simulink model "final_lqr_integral_nonlinear_simulation"  (R2024a)
settings: Solver=VariableStepAuto  StartTime=0.0  StopTime=10.0  RelTol=1e-3
undefined symbols (not defined in the file): g_val, Ki, Kx, m_val, r_pos
libraries: slpidlib x1
settings Model: Creator=yufon  LastModifiedBy=yufon

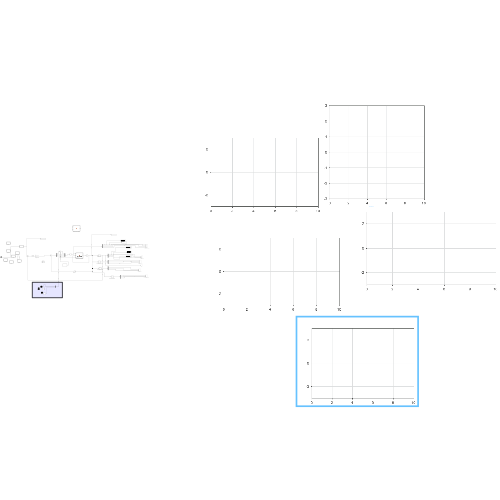
[thumbnail: Simulink's stored preview of the top-level diagram]
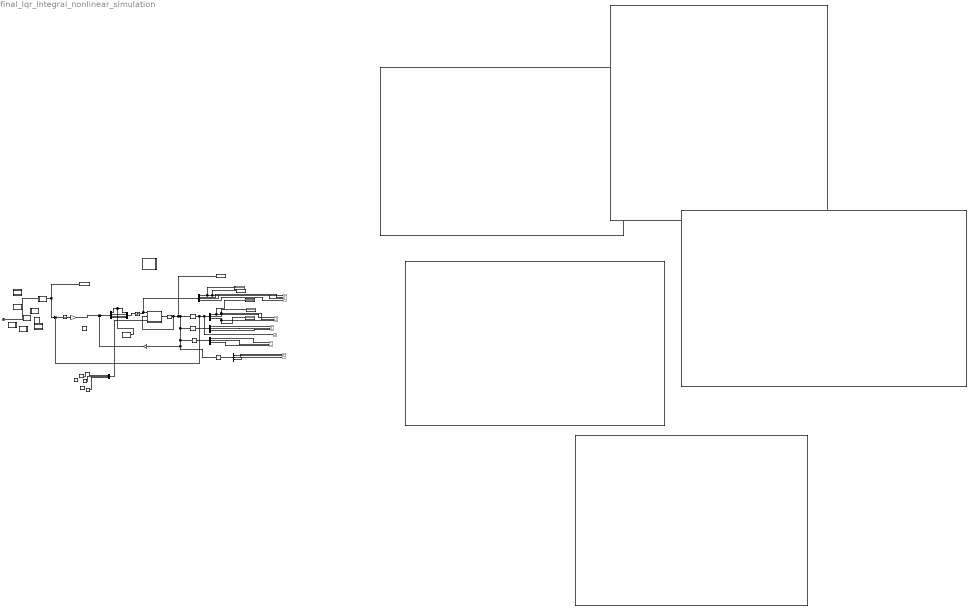
== system final_lqr_integral_nonlinear_simulation ==
  note: Wind Purtubabtions
  Arc : MATLAB Function  TreatAsAtomicUnit=on
  Body Abgular Selector : Selector  InputPortWidth=12  IndexOptions=Index vector (dialog)  Indices=[10 11 12]  OutputSizes=1
  Body Abgular Selector1 : Selector  InputPortWidth=12  IndexOptions=Index vector (dialog)  Indices=[7 8 9]  OutputSizes=1
  Body Linear Velocities : Scope  Commented=on  NumInputPorts=3
  Circular Trajectory : MATLAB Function  TreatAsAtomicUnit=on
  Clock : Clock
  Constant1 : Constant  Value=r_pos  VectorParams1D=off
  Constant2 : Constant  Value=m_val*g_val
  Constant4 : Constant  Value=0
  Constant5 : Constant  Value=0
  Control Input Scope : Scope  Commented=on  NumInputPorts=4
  Dashboard Scope{,1..4} (5 alike) : DashboardScope
  Demux{,1,3,5} (4 alike) : Demux  Outputs=3
  Demux2 : Demux
  Demux6 : Demux
  Display{,1..3} (4 alike) : Display
  Figure 8 : MATLAB Function  TreatAsAtomicUnit=on
  Helical : MATLAB Function  TreatAsAtomicUnit=on
  Integrator Gain : Gain  Gain=Ki  Multiplication=Matrix(K*u)
  Integrator4 : Integrator  InitialCondition=[0; 0; 0; zeros(9,1)]
  Integrator5 : Integrator
  LQR Gain : Gain  Gain=Kx  Multiplication=Matrix(K*u)
  Line : MATLAB Function  TreatAsAtomicUnit=on
  MATLAB Function1 : MATLAB Function  TreatAsAtomicUnit=on
  Mux2 : Mux
  Mux3 : Mux  Inputs=3
  Orientation Scope : Scope  Commented=on  NumInputPorts=3
  Orientation Selector1 : Selector  InputPortWidth=12  IndexOptions=Index vector (dialog)  Indices=[4 5 6]  OutputSizes=1
  PID Controller : slpidlib/PID Controller  Controller=PID  Form=Parallel  TimeDomain=Continuous-time  UseExternalTs=off  SampleTime=-1  IntegratorMethod=Forward Euler  FilterMethod=Forward Euler  ControllerParametersSource=internal  P=1  I=1  UseKiTs=off  D=0  UseExternalDerivativeSource=off  N=100  UseFilter=on  TunerSelectOption=Transfer Function Based (PID Tuner App)  InitialConditionSource=internal  InitialConditionForIntegrator=0  InitialConditionForFilter=0  DifferentiatorICPrevScaledInput=0  ExternalReset=none  TrackingMode=off  Kt=1  LimitOutput=off  SatLimitsSource=internal  UpperSaturationLimit=inf  LowerSaturationLimit=-inf  LinearizeAsGain=on  AntiWindupMode=none  Kb=1  LimitIntegrator=off  UpperIntegratorSaturationLimit=inf  LowerIntegratorSaturationLimit=-inf  POutMin=[]  POutMax=[]  IOutMin=[]  IOutMax=[]  DOutMin=[]  DOutMax=[]  NOutMin=[]  NOutMax=[]  SumOutMin=[]  SumOutMax=[]  SaturationOutMin=[]  SaturationOutMax=[]  PParamMin=[]  PParamMax=[]  IParamMin=[]  IParamMax=[]  DParamMin=[]  DParamMax=[]  NParamMin=[]  NParamMax=[]  KbParamMin=[]  KbParamMax=[]  KtParamMin=[]  KtParamMax=[]  KbOutMin=[]  KbOutMax=[]  KtOutMin=[]  KtOutMax=[]  IntegratorOutMin=[]  IntegratorOutMax=[]  FilterOutMin=[]  FilterOutMax=[]  SumI1OutMin=[]  SumI1OutMax=[]  SumI2OutMin=[]  SumI2OutMax=[]  SumI3OutMin=[]  SumI3OutMax=[]  SumI4OutMin=[]  SumI4OutMax=[]  SumDOutMin=[]  SumDOutMax=[]  DifferentiatorOutMin=[]  DifferentiatorOutMax=[]  FilterDiffOutCoefMin=[]  FilterDiffOutCoefMax=[]  ReciprocalOutMin=[]  ReciprocalOutMax=[]  SumDenOutMin=[]  SumDenOutMax=[]  SumNumOutMin=[]  SumNumOutMax=[]  DivideOutMin=[]  DivideOutMax=[]  UdiffTsProdOutMin=[]  UdiffTsProdOutMax=[]  NTsProdOutMin=[]  NTsProdOutMax=[]  UintegralTsProdOutMin=[]  UintegralTsProdOutMax=[]  UngainTsProdOutMin=[]  UngainTsProdOutMax=[]  ClampingZeroOutDataTypeStr=Inherit: Inherit via back propagation  ClampingZeroOutMin=[]  ClampingZeroOutMax=[]  FilterDenConstantOutDataTypeStr=Inherit: Inherit via back propagation  FilterDenConstantOutMin=[]  FilterDenConstantOutMax=[]  PCopyOutDataTypeStr=Inherit: Inherit via back propagation  PCopyOutMin=[]  PCopyOutMax=[]  NCopyOutDataTypeStr=Inherit: Inherit via back propagation  NCopyOutMin=[]  NCopyOutMax=[]  IntegratorContinuousStateAttributes=''  IntegratorStateMustResolveToSignalObject=off  IntegratorRTWStateStorageClass=Auto  FilterContinuousStateAttributes=''  FilterStateMustResolveToSignalObject=off  FilterRTWStateStorageClass=Auto  ParallelPVariant=InternalParameters  IdealPVariant=Disabled  IVariant=InternalParameters  DVariant=InternalParameters  IntegratorVariant=Continuous  SatVariant=Disabled  AWVariant=Passthrough  PCopyVariant=Disabled  TRVariant=Disabled  FdbkBlocksVariant=Forward  IdealPFdbkVariant=Disabled  SatFdbkVariant=Disabled  DerivativeFilterVariant=ContFilter  NVariant=InternalParameters  NCopyVariant=Disabled  FilterICVariant=InternalICsFilter  IntegratorICVariant=InternalICs  ExternalResetVariant=Disabled  TRSumVariant=Passthrough  SumFdbkVariant=Disabled  SumVariant=Sum_PID  TsampFilterVariant=InternalTs  TsampNgainVariant=Passthrough  TsampIntegralVariant=Disabled_SignalSpec  ExternalSaturationOutDataTypeStr=Inherit: Same as second input  DerivativeSourceVariant=ErrorSignal
  Position Scope : Scope  Commented=on  NumInputPorts=3
  Position Scope1 : Scope  Commented=on  NumInputPorts=3
  Position Selector : Selector  InputPortWidth=12  IndexOptions=Index vector (dialog)  Indices=[1 2 3]  OutputSizes=1
  Pulse Generator1 : DiscretePulseGenerator  Amplitude=10  Period=10  PulseWidth=5  PhaseDelay=20  SampleTime=10
  Pulse Generator3 : DiscretePulseGenerator  PulseType=Time based  Amplitude=3  Period=5  PhaseDelay=100
  Pulse Generator4 : DiscretePulseGenerator  PulseType=Time based  Amplitude=3  Period=10  PulseWidth=5  PhaseDelay=50
  Quadrotor Nonlinear Model1 : MATLAB Function  TreatAsAtomicUnit=on
  Quadrotor Nonlinear Model2 : MATLAB Function  TreatAsAtomicUnit=on
  Saturation1 : Saturate  UpperLimit=[40; 0.15; 0.1;0.1]  LowerLimit=[0; -0.15; -0.10; -0.10]
  Scope : Scope  Commented=on
  Simusoidal : MATLAB Function  TreatAsAtomicUnit=on
  Spiral : MATLAB Function  TreatAsAtomicUnit=on
  Sum : Sum  Inputs=|--
  Sum1 : Sum  Inputs=|+-
  Sum3 : Sum  Inputs=|++
  To Workspace : ToWorkspace  VariableName=X_states  SampleTime=-1
  To Workspace1 : ToWorkspace  VariableName=U1  SaveFormat=Timeseries  SampleTime=-1
  To Workspace2 : ToWorkspace  VariableName=r_traj  SaveFormat=Timeseries  SampleTime=-1
  wires:
  Constant4/1 -> Mux3/2
  Demux3/1 -> Position Scope1/1  "p"
  Saturation1/1 -> Demux2/1, Quadrotor Nonlinear Model1/1(u)
  Orientation Selector1/1 -> Demux1/1
  Pulse Generator4/1 -> Mux3/1
  Demux1/1 -> Orientation Scope/1  "Phi"
  Clock/1 -> MATLAB Function1/1(t)
  Constant5/1 -> Mux3/3
  Demux5/3 -> Body Linear Velocities/3  "w"
  Demux1/2 -> Orientation Scope/2  "Thata"
  Integrator Gain/1 -> Sum/1
  Sum1/1 -> Integrator5/1
  Demux6/1 -> Sum3/1  "U1"
  Sum3/1 -> Mux2/1
  Quadrotor Nonlinear Model1/1(dx) -> Integrator4/1  "X_states"
  Demux/3 -> Display1/1, Position Scope/3  "Z"
  Demux3/2 -> Position Scope1/2  "q"
  Demux2/1 -> Display3/1, To Workspace1/1, Control Input Scope/1  "U1"
  Demux1/3 -> Orientation Scope/3  "Psi"
  Demux3/3 -> Position Scope1/3  "r"
  MATLAB Function1/1(r) -> To Workspace2/1, Sum1/1
  Demux/1 -> Display2/1, Position Scope/1  "X"
  Demux6/3 -> Mux2/3  "U3"
  Integrator4/1 -> To Workspace/1, Body Abgular Selector1/1, LQR Gain/1, Body Abgular Selector/1, Orientation Selector1/1, Position Selector/1, Quadrotor Nonlinear Model1/2(x)
  Mux3/1 -> Quadrotor Nonlinear Model1/3(F_wind_body)
  Demux2/2 -> Control Input Scope/2  "U2"
  Body Abgular Selector/1 -> Demux3/1
  Demux2/3 -> Control Input Scope/3  "U3"
  Position Selector/1 -> Scope/1, Demux/1, Sum1/2
  Demux6/4 -> Mux2/4  "U4"
  Mux2/1 -> Saturation1/1
  Constant2/1 -> Sum3/2
  Demux/2 -> Display/1, Position Scope/2  "Y"
  LQR Gain/1 -> Sum/2
  Demux2/4 -> Control Input Scope/4  "U4"
  Demux5/2 -> Body Linear Velocities/2  "u"
  Demux6/2 -> Mux2/2  "U2"
  Body Abgular Selector1/1 -> Demux5/1
  Integrator5/1 -> Integrator Gain/1
  Sum/1 -> Demux6/1
  Demux5/1 -> Body Linear Velocities/1  "u"

== matlab function final_lqr_integral_nonlinear_simulation/Line ==
  data: t input; r output
function r = linear_ref(t)
    % Define total time and start/end positions
    T_total = 50;  % duration of trajectory
    r_start = [0; 0; 0];
    r_end   = [5; 5; 5];

    % Clamp progress between 0 and 1
    progress = min(max(t / T_total, 0), 1);

    % Linear interpolation
    r = r_start + (r_end - r_start) * progress;
end

== matlab function final_lqr_integral_nonlinear_simulation/MATLAB Function1 ==
  data: t input; r output
function r = rectangular_trajectory(t)
    % Rectangular trajectory parameters
    x_length = 10;       % Rectangle length (x-direction) in meters
    y_width = 8;         % Rectangle width (y-direction) in meters
    z_height = 5;        % Z height in meters
    duration = 500;       % Total duration in seconds
    
    % Add initial offset to match quadcopter starting position
    x_offset = 0;        % Starting at x=0
    y_offset = 0;        % Starting at y=0
    z_offset = 0;        % Starting at z=0
    
    % Time progression (clamped between 0 and 1)
    progress = min(max(t / duration, 0), 1);
    
    % Define the four segments of the rectangle
    % Each segment takes 25% of the total time
    if progress < 0.25 
        % First segment: Moving along x-axis (0 to x_length)
        segment_progress = progress / 0.25;
        x_ref = x_offset + x_length * segment_progress;
        y_ref = y_offset;
        z_ref = z_offset + z_height * segment_progress;
    elseif progress < 0.5
        % Second segment: Moving along y-axis (0 to y_width)
        segment_progress = (progress - 0.25) / 0.25;
        x_ref = x_offset + x_length;
        y_ref = y_offset + y_width * segment_progress;
        z_ref = z_offset + z_height;
    elseif progress < 0.75
        % Third segment: Moving along x-axis (x_length to 0)
        segment_progress = (progress - 0.5) / 0.25;
        x_ref = x_offset + x_length * (1 - segment_progress);
        y_ref = y_offset + y_width;
        z_ref = z_offset + z_height;
    else
        % Fourth segment: Moving along y-axis (y_width to 0)
        segment_progress = (progress - 0.75) / 0.25;
        x_ref = x_offset;
        y_ref = y_offset + y_width * (1 - segment_progress);
        z_ref = z_offset + z_height;
    end
    
    r = [x_ref; y_ref; z_ref];
end

== matlab function final_lqr_integral_nonlinear_simulation/Quadrotor Nonlinear Model1 ==
  data: u input size=[4 1]; x input size=[12 1]; dx output size=[12 1]; F_wind_body input
function dx = quadrotor_dynamics(u, x, F_wind_body)
    % Physical parameters
    m = 0.547; % Mass [kg]
    g = 9.81; % Gravity [m/s^2]
    Cd = 1.0; % Drag coefficient [-]
    Ix = 3.3e-3;
    Iy = 3.3e-3;
    Iz = 5.8e-3;
    Ax = 0.011;
    Ay = 0.011;
    Az = 0.022;
    rho = 1.225; % Air density [kg/m^3]
    
    % REMOVE THIS LINE - it overwrites the input state!
    % x = zeros(12,1);
    
    % State unpacking
    phi = x(4); theta = x(5); psi = x(6);
    u_b = x(7); v_b = x(8); w_b = x(9);
    p = x(10); q = x(11); r = x(12);


    % Compute wind acceleration
    a_wind_body = F_wind_body / m;
    
    % Input unpacking with saturation
    U1 = max(0, min(30*m*g, u(1))); % Limit thrust to reasonable bounds
    U2 = max(-10, min(10, u(2)));   % Limit torques
    U3 = max(-10, min(10, u(3)));
    U4 = max(-10, min(10, u(4)));
    
    % Trig functions
    s = @sin; c = @cos; t = @tan;
    
    % Safety factor to prevent division by zero or extreme values
    eps = 1e-4;
    safe_cos_theta = max(eps, abs(cos(theta)));
    
    dx = zeros(12,1);
    
    % Translational Kinematics (Inertial frame)
    dx(1) = u_b*(c(theta)*c(psi)) + v_b*(s(phi)*s(theta)*c(psi) - c(phi)*s(psi)) + w_b*(c(phi)*s(theta)*c(psi) + s(phi)*s(psi));
    dx(2) = u_b*(c(theta)*s(psi)) + v_b*(s(phi)*s(theta)*s(psi) + c(phi)*c(psi)) + w_b*(c(phi)*s(theta)*s(psi) - s(phi)*c(psi));
    dx(3) = -u_b*s(theta) + v_b*s(phi)*c(theta) + w_b*c(phi)*c(theta);
    
    % Rotational Kinematics - with singularity protection
    if abs(theta) > 0.95*pi/2
        % Near singularity - limit change
        dx(4) = p;
        dx(5) = c(phi)*q - s(phi)*r;
        dx(6) = 0;
    else
        dx(4) = p + s(phi)*t(theta)*q + c(phi)*t(theta)*r;
        dx(5) = c(phi)*q - s(phi)*r;
        dx(6) = s(phi)/safe_cos_theta*q + c(phi)/safe_cos_theta*r;
    end
    
    % Translational Dynamics (Body frame)
    dx(7) = g*s(theta) - q*w_b + r*v_b - (rho*Cd*Ax*u_b*abs(u_b))/(2*m) + a_wind_body(1);
    dx(8) = -g*c(theta)*s(phi) - r*u_b + p*w_b - (rho*Cd*Ay*v_b*abs(v_b))/(2*m) + a_wind_body(2);
    dx(9) = -g*c(theta)*c(phi) + U1/m - p*v_b + q*u_b - (rho*Cd*Az*w_b*abs(w_b))/(2*m) + a_wind_body(3);
    
    % Rotational Dynamics
    dx(10) = (U2 + (Iy - Iz)*q*r)/Ix;
    dx(11) = (U3 + (Iz - Ix)*r*p)/Iy;
    dx(12) = (U4 + (Ix - Iy)*p*q)/Iz;
end

== matlab function final_lqr_integral_nonlinear_simulation/Quadrotor Nonlinear Model2 ==
  data: u input size=[4 1]; x input size=[12 1]; dx output size=[12 1]
function dx = quadrotor_dynamics(u, x)
% Inputs:
%   t   - time (optional, use [] if unused)
%   x   - 12x1 state vector [x; y; z; phi; theta; psi; u; v; w; p; q; r]
%   u   - 4x1 control inputs [U1; U2; U3; U4]
%   m,g,rho,Cd,Ax,Ay,Az,Ix,Iy,Iz - physical parameters


% x = [x; y; z; phi; theta; psi; u; v; w; p; q; r]
% Position (inertial): x(1:3)
% Orientation (Euler): x(4:6)
% Linear velocity (body): x(7:9)
% Angular velocity (body): x(10:12)


% Quadcopter Physical Constants
m     = 0.547;                 % Mass [kg]
g     = 9.81;                  % Gravity [m/s^2]
% L     = 0.17;                  % Arm length [m]
% kF    = 1.5e-7;                % Thrust coefficient [N/RPM^2]
% kM    = 3.75e-7;               % Torque coefficient [Nm/RPM^2]
Cd    = 1.0;                   % Drag coefficient [-]

% Inertia matrix components [kg*m^2]
Ix    = 3.3e-3;
Iy    = 3.3e-3;
Iz    = 5.8e-3;

% Cross-sectional areas [m^2]
Ax    = 0.011;
Ay    = 0.011;
Az    = 0.022;

% Air density (if needed for aerodynamic forces)
rho   = 1.225;  % Air density at sea level [kg/m^3]
x = zeros(12,1);


% Outputs:
%   dx - 12x1 derivative of states

% State unpacking
phi   = x(4); theta = x(5); psi = x(6);
u_b = x(7);  v_b = x(8);  w_b = x(9);
p   = x(10); q   = x(11); r   = x(12);

% Input unpacking
U1 = u(1); U2 = u(2); U3 = u(3); U4 = u(4);

% Rotation helpers
s = @sin; c = @cos; t = @tan;

% Output
%x = zeros(12,1);
dx = zeros(12,1);   % Explicitly declare dx as a 12x1 column vector


% Translational Kinematics (Inertial frame)
dx(1) = u_b*(c(theta)*c(psi)) + v_b*(s(phi)*s(theta)*c(psi) - c(phi)*s(psi)) + w_b*(c(phi)*s(theta)*c(psi) + s(phi)*s(psi));
dx(2) = u_b*(c(theta)*s(psi)) + v_b*(s(phi)*s(theta)*s(psi) + c(phi)*c(psi)) + w_b*(c(phi)*s(theta)*s(psi) - s(phi)*c(psi));
dx(3) = -u_b*s(theta) + v_b*s(phi)*c(theta) + w_b*c(phi)*c(theta);

% Rotational Kinematics
dx(4) = p + s(phi)*t(theta)*q + c(phi)*t(theta)*r;
dx(5) = c(phi)*q - s(phi)*r;
dx(6) = s(phi)/c(theta)*q + c(phi)/c(theta)*r;

% Translational Dynamics (Body frame)
dx(7) = g*s(theta) - q*w_b + r*v_b - (rho*Cd*Ax*u_b*abs(u_b))/(2*m + 1e-6);
dx(8) = -g*c(theta)*s(phi) - r*u_b + p*w_b - (rho*Cd*Ay*v_b*abs(v_b))/(2*m + 1e-6);
dx(9) = -g*c(theta)*c(phi) + U1/m - p*v_b + q*u_b - (rho*Cd*Az*w_b*abs(w_b))/(2*m + 1e-6);

% Rotational Dynamics
dx(10) = (U2 + (Iy - Iz)*q*r)/Ix;
dx(11) = (U3 + (Iz - Ix)*r*p)/Iy;
dx(12) = (U4 + (Ix - Iy)*p*q)/Iz;

end

== matlab function final_lqr_integral_nonlinear_simulation/Arc ==
  data: t input; r output
function r = arc_trajectory(t)
    % Arc parameters
    R = 5;
    theta_start = 0;
    theta_end = pi/2;
    duration = 10;
    z_const = 5;
    
    % Add initial offset to match quadcopter starting position
    x_offset = 0;  % Starting at x=0
    y_offset = 0;  % Starting at y=0
    z_offset = 0;  % Starting at z=0
    
    % Time progression
    progress = min(max(t / duration, 0), 1);
    theta = theta_start + progress * (theta_end - theta_start);
    
    % Reference position with offset
    x_ref = x_offset + (R * cos(theta) - R * cos(theta_start)) * progress;
    y_ref = y_offset + (R * sin(theta) - R * sin(theta_start)) * progress;
    z_ref = z_offset + z_const * progress;
    
    r = [x_ref; y_ref; z_ref];
end

== matlab function final_lqr_integral_nonlinear_simulation/Simusoidal ==
  data: t input; r output
function r = sinusoidal_trajectory(t)
    % Sinusoidal trajectory with varying frequencies
    % Parameters
    x_amp = 5;           % X amplitude in meters
    y_amp = 3;           % Y amplitude in meters
    z_max = 5;           % Maximum z height in meters
    duration = 500;       % Total duration in seconds
    
    % Frequency parameters
    f_start = 0.1;       % Starting frequency in Hz
    f_end = 0.5;         % Ending frequency in Hz
    
    % Add initial offset to match quadcopter starting position
    x_offset = 0;        % Starting at x=0
    y_offset = 0;        % Starting at y=0
    z_offset = 0;        % Starting at z=0
    
    % Time progression (clamped between 0 and 1)
    progress = min(max(t / duration, 0), 1);
    
    % Varying frequency over time (linear interpolation)
    current_freq = f_start + progress * (f_end - f_start);
    
    % Phase shift to ensure y is 90 degrees out of phase with x
    phase_shift = pi/2;
    
    % Calculate positions
    x_ref = x_offset + x_amp * sin(2 * pi * current_freq * t);
    y_ref = y_offset + y_amp * sin(2 * pi * current_freq * t + phase_shift);
    z_ref = z_offset + z_max * progress;
    
    r = [x_ref; y_ref; z_ref];
end

== matlab function final_lqr_integral_nonlinear_simulation/Spiral ==
  data: t input; r output
function r = spiral_trajectory(t)
    % Spiral Trajectory Generator

    % Parameters
    R = 5;                 % Radius of spiral (constant)
    duration = 500;         % Total time for spiral traversal
    turns = 2;             % Number of full 2π turns
    height = 5;            % Total height climbed

    % Time normalization
    progress = min(max(t / duration, 0), 1);

    % Angle progresses from 0 to 2π * turns
    theta = progress * (2 * pi * turns);

    % Spiral path in x, y and ascending in z
    x_ref = R * cos(theta);
    y_ref = R * sin(theta);
    z_ref = height * progress;

    % Output reference position
    r = [x_ref; y_ref; z_ref];
end

== matlab function final_lqr_integral_nonlinear_simulation/Figure 8 ==
  data: t input; r output
function r = figure_eight_trajectory(t)
    % Parameters
    R = 5;               % Radius of the loops
    omega = 0.2;         % Angular speed [rad/s]
    duration = 500;       % Total time to complete one figure-eight
    z_const = 5;         % Constant height
    
    % Initial offset (optional)
    x_offset = 0;
    y_offset = 0;
    z_offset = 0;

    % Time progression
    progress = min(max(t / duration, 0), 1);
    theta = omega * t;

    % Figure-eight Lissajous shape
    x_ref = x_offset + R * sin(theta);
    y_ref = y_offset + R * sin(theta) .* cos(theta);
    z_ref = z_offset + z_const;

    r = [x_ref; y_ref; z_ref];
end

== matlab function final_lqr_integral_nonlinear_simulation/Helical ==
  data: t input; r output
function r = helical_trajectory(t)
    % Parameters
    R = 5;              % Radius in meters
    omega = 2 * pi / 20; % Angular speed (rad/s) for smooth loops
    z_max = 10;         % Max height
    duration = 500;     % Total trajectory time in seconds

    % Time progress normalized
    progress = min(max(t / duration, 0), 1);
    theta = omega * t;

    % Reference position, offset to start at (0, 0, 0)
    x_ref = R * (cos(theta) - 1);   % cos(0) - 1 = 0
    y_ref = R * sin(theta);
    z_ref = z_max * progress;

    r = [x_ref; y_ref; z_ref];
end

== matlab function final_lqr_integral_nonlinear_simulation/Circular Trajectory ==
  data: t input; r output


function r = trajectory(t)

% Parameters (you can also pass these in or make them tunable)
R = 5;           % Radius of circle (meters)
omega = 0.1;     % Angular frequency (rad/s)
z0 = 10;         % Base altitude (meters)
A = 2;           % Amplitude of vertical oscillation (meters)
omega_z = 0.05;  % Vertical oscillation frequency (rad/s)


x_offset = 0;  % Starting at x=0
y_offset = 0;  % Starting at y=0
z_offset = 0;  % Starting at z=0

% Reference trajectory components
r_x =x_offset + R * cos(omega * t);
r_y =y_offset + R * sin(omega * t);
r_z = z_offset + z0 + 0 * sin(omega_z * t);  % Set A = 0 for pure circle

% Output as a 3x1 vector
r = [r_x; r_y; r_z];
